simulink model "Test_N9"  (R2020b)
settings: Solver=ode3  StartTime=0.0  StopTime=inf  FixedStep=0.05  RelTol=1e-3
libraries: Utilities x2, XBotBlockToolbox x2

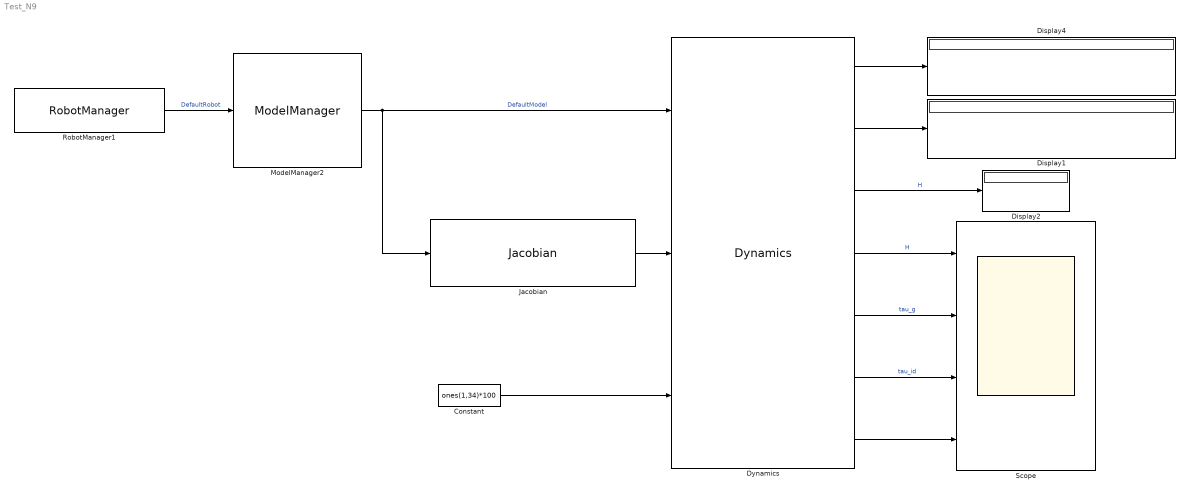
== system Test_N9 ==
  Constant : Constant  Value=ones(1,34)*100
  Display1 : Display
  Display2 : Display
  Display4 : Display
  Dynamics : Utilities/Dynamics  ModelName=DefaultModel  ComponentsList={ 'B', 'BInv', 'M', 'H', 'tau_g', 'tau_id', 'tau_id_const' }
  Jacobian : Utilities/Jacobian  ModelName=DefaultModel  JacobianList={ 'J' }  LinkName=torso  ExternalRef=Off  TargetLink=LWrMot3  BaseLink=LWrMot2
  ModelManager2 : XBotBlockToolbox/ModelManager  ModelName=DefaultModel  RobotName=DefaultRobot  UseExtModel=Off  SyncWithRobot=On  GetFloatingBaseList={}  SetFloatingBaseComponent=Off  GravityRequest=Off  ReadingsList={}  MechanicalLimitsList={}  MechanicalLimitsCheck=Off  MechanicalLimitsEnforce=Off  SensorList={}  ReferencesList={}  OldModelName=DefaultModel
  RobotManager1 : XBotBlockToolbox/RobotManager  RobotName=DefaultRobot  ModelName=DefaultModel  UseExtRobot=Off  SyncWithModel=Off  ReadingsList={}  MechanicalLimitsList={}  MechanicalLimitsCheck=Off  MechanicalLimitsEnforce=Off  SensorList={}  ReferencesList={}  OldRobotName=DefaultRobot
  Scope : Scope  NumInputPorts=4
  wires:
  RobotManager1/1 -> ModelManager2/1  "DefaultRobot"
  ModelManager2/1 -> Dynamics/1, Jacobian/1  "DefaultModel"
  Dynamics/1 -> Display4/1
  Dynamics/4 -> Scope/1  "H"
  Dynamics/5 -> Scope/2  "tau_g"
  Dynamics/6 -> Scope/3  "tau_id"
  Dynamics/2 -> Display1/1
  Jacobian/1 -> Dynamics/2
  Constant/1 -> Dynamics/3
  Dynamics/7 -> Scope/4
  Dynamics/3 -> Display2/1  "H"
